simulink model "Schema_Commande"  (R2025b)
settings: Solver=VariableStepAuto  StartTime=0.0  StopTime=10.0  RelTol=1e-3
settings Model: Creator=Louis  LastModifiedBy=Louis

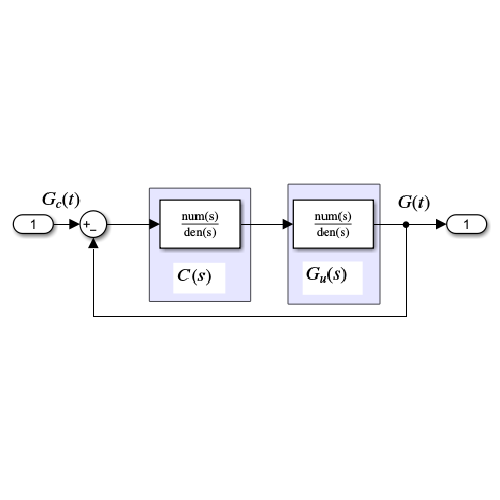
[thumbnail: Simulink's stored preview of the top-level diagram]
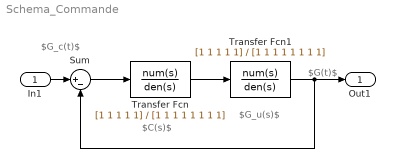
== system Schema_Commande ==
  note: $G_u(s)$
  note: $C(s)$
  note: $G(t)$
  note: $G_c(t)$
  In1 : Inport
  Sum : Sum  Inputs=|+-
  Transfer Fcn : TransferFcn  Numerator=[1 1 1 1 1]  Denominator=[1 1 1 1 1 1 1 1]
  Transfer Fcn1 : TransferFcn  Numerator=[1 1 1 1 1]  Denominator=[1 1 1 1 1 1 1 1]
  Out1 : Outport
  wires:
  Sum/1 -> Transfer Fcn/1
  Transfer Fcn/1 -> Transfer Fcn1/1
  Transfer Fcn1/1 -> Out1/1, Sum/2
  In1/1 -> Sum/1
